simulink model "pure_pursuit"  (R2018a)
settings: Solver=VariableStepAuto  StartTime=0.0  StopTime=8  RelTol=1e-3
libraries: simulink x1, roblocks x1, simulink_need_slupdate x1
settings Model: Creator=Admin  LastModifiedBy=Admin

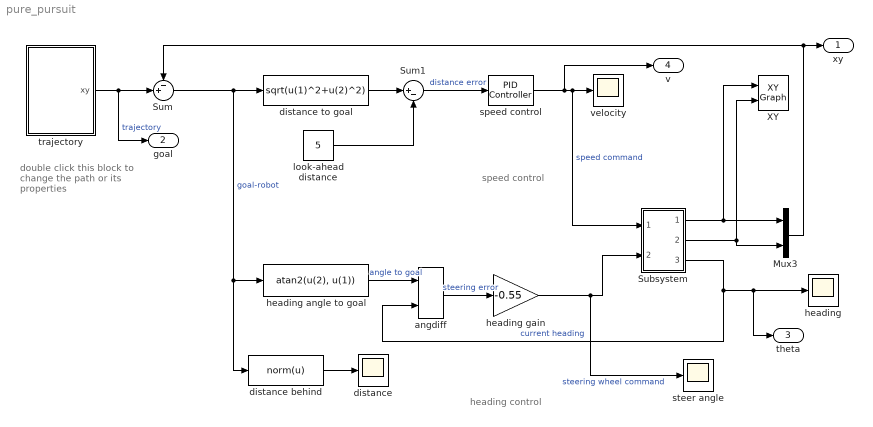
== system pure_pursuit ==
  note: double click this block to
      | change the path or its
      | properties
  note: heading control
  note: speed control
  Mux3 : Mux  Inputs=2
  Subsystem : Subsystem
  Sum : Sum  Inputs=-+|
  Sum1 : Sum  Inputs=|+-
  XY : simulink/Sinks/XY Graph  xmin=0  xmax=15  ymin=0  ymax=15  st=-1
  angdiff : roblocks/Toolbox/angdiff
  distance : Scope
  distance behind : MATLABFcn  MATLABFcn=norm(u)
  distance to goal : Fcn  Expr=sqrt(u(1)^2+u(2)^2)
  "heading " : Scope
  heading angle to goal : Fcn  Expr=atan2(u(2), u(1))
  heading gain : Gain  Gain=-0.55
  look-ahead distance : Constant  Value=5
  speed control : simulink_need_slupdate/PID Controller  P=0.2  I=3  D=0
      settings: SourceProductName=Simulink
  steer angle : Scope
  trajectory : Subsystem  mask(Trajectory generator){path=|, vaxis=[2.0 2.0], tseg=[], dt=0.1, tacc=0, setsimtime=on}
      mask path=|
      | [ 4 4;
      |  8 7;
      |  12 4;
      |  4 4 ]
      mask prompts: vaxis "Axis velocities"; tseg "Segment times"; dt "Sample interval"; tacc "Acceleration time"; setsimtime "Set Simulink simulation time"
      mask help: Generate an n-dimensional trajectory using the Toolbox function mstraj.
      mask init:
      | robot_traj = mstraj(path(2:end,:), vaxis, tseg, path(1,:), dt, tacc);
      | total_time = size(robot_traj,1)*dt;
      | if setsimtime
      |     set_param(gcs, 'StopTime', num2str(total_time));
      | end
      mask Help:
      | The trajectory requires a number of parameters
      | 
      | Path: an MxN matrix that defines a path with M points (start, intermediate, goal) and each point is defined by an N-dimensional vector.
      | 
      | Axis velocities: a 1xM vector that specifies the maximum speed of each motion for each dimension.
      | 
      | Segment times: a 1x(N-1) vector of times to execute each motion segment.
      | 
      | Sample time: a scalar sampling time, the trajectory is computed at discrete times with this separation.
      | 
      | Acceleration time: a scalar giving the period of acceleration at each waypoint, as the motion accelerates from one segment to the next.  Can be zero.
      | 
      | This block sets the Simulink simulation time to the length of the trajectory.
      mask Display: plot(path(:,1), path(:,2))
  velocity : Scope
  xy : Outport
  goal : Outport  Port=2
  theta : Outport  Port=3
  v : Outport  Port=4
  wires:
  Sum/1 -> distance behind/1, heading angle to goal/1, distance to goal/1  "goal-robot"
  look-ahead distance/1 -> Sum1/2
  speed control/1 -> Subsystem/1(In1), velocity/1, v/1  "speed command"
  Subsystem/2(Out2) -> Mux3/2, XY/2
  heading gain/1 -> steer angle/1, Subsystem/2(In2)  "steering wheel command"
  Mux3/1 -> Sum/1, xy/1
  distance to goal/1 -> Sum1/1
  trajectory/1(xy) -> goal/1, Sum/2  "trajectory"
  heading angle to goal/1 -> angdiff/1  "angle to goal"
  Sum1/1 -> speed control/1  "distance error"
  angdiff/1 -> heading gain/1  "steering error"
  distance behind/1 -> distance/1
  Subsystem/3(Out3) -> "heading "/1, theta/1, angdiff/2  "current heading"
  Subsystem/1(Out1) -> Mux3/1, XY/1

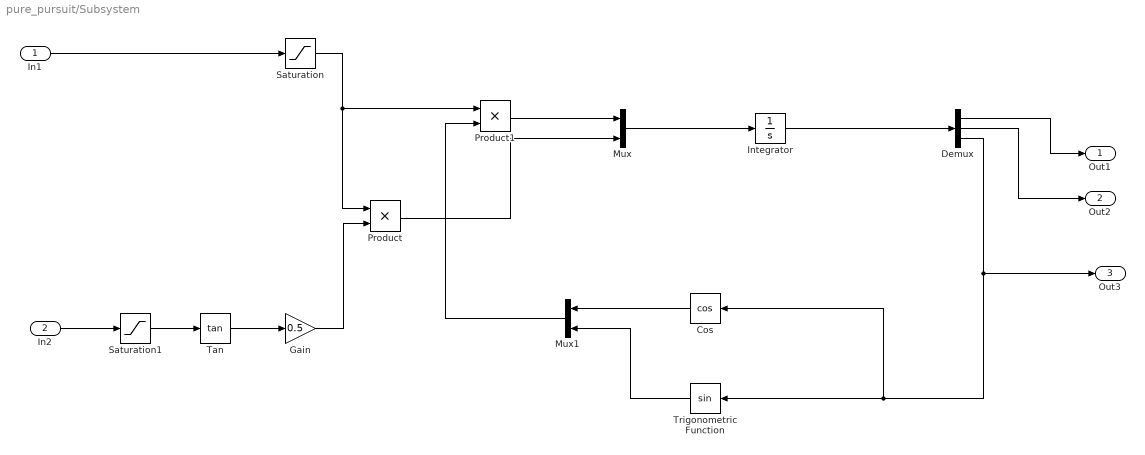
== system pure_pursuit/Subsystem ==
  In1 : Inport
  In2 : Inport  Port=2
  Cos : Trigonometry  Operator=cos
  Demux : Demux  Outputs=3
  Gain : Gain  Gain=0.5
  Integrator : Integrator
  Mux : Mux  Inputs=2
  Mux1 : Mux  Inputs=2
  Product : Product
  Product1 : Product
  Saturation : Saturate  UpperLimit=2.5  LowerLimit=-2.5
  Saturation1 : Saturate  UpperLimit=2*pi/3  LowerLimit=-2*pi/3
  Tan : Trigonometry  Operator=tan
  Trigonometric Function : Trigonometry
  Out1 : Outport
  Out2 : Outport  Port=2
  Out3 : Outport  Port=3
  wires:
  Demux/3 -> Out3/1, Cos/1, Trigonometric Function/1
  Mux1/1 -> Product1/2
  Product1/1 -> Mux/1
  Saturation/1 -> Product/1, Product1/1
  Demux/2 -> Out2/1
  Product/1 -> Mux/2
  Gain/1 -> Product/2
  Integrator/1 -> Demux/1
  Tan/1 -> Gain/1
  Mux/1 -> Integrator/1
  Saturation1/1 -> Tan/1
  Cos/1 -> Mux1/1
  Trigonometric Function/1 -> Mux1/2
  In1/1 -> Saturation/1
  In2/1 -> Saturation1/1
  Demux/1 -> Out1/1

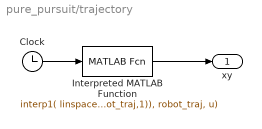
== system pure_pursuit/trajectory ==
  Clock : Clock
  Interpreted MATLAB Function : MATLABFcn  MATLABFcn=interp1( linspace(0, total_time, size(robot_traj,1)), robot_traj, u)
  xy : Outport
  wires:
  Clock/1 -> Interpreted MATLAB Function/1
  Interpreted MATLAB Function/1 -> xy/1
